simulink model "ModeStatAndRsp"  (R2018b)
settings: Solver=FixedStepDiscrete  StartTime=0.0  StopTime=10.0  FixedStep=0.01  RelTol=1e-3
undefined symbols (not defined in the file): c_RecvL, c_RecvLR, c_RecvR, IfVeSMSeStNumConfig, KeSMSbMdChime2Enable_Val, KeSMSbSRSPosNumConfig_Val, KeSMSuChmReqDurnTm_Val, KeSMSuChmReqIntlTm_Val, KeSMSuRspStatHldTm_Val, MdRspLocal1, MdTp1, ModeNum, PowerMode1, SrcReqTp1, srsconvert
libraries: RspLib x47, simulink x1
(part 7 of 8)

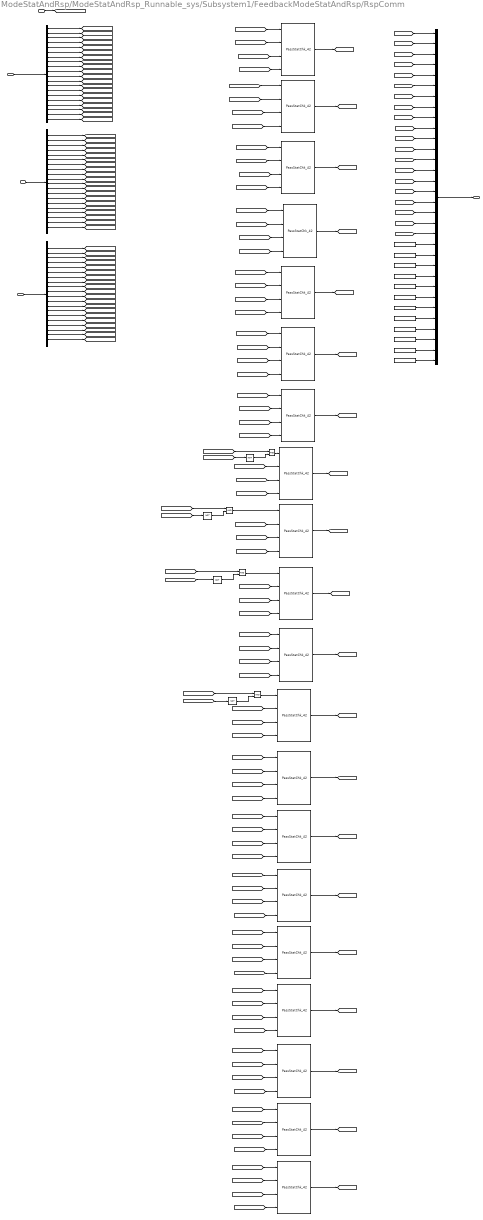
== system ModeStatAndRsp/ModeStatAndRsp_Runnable_sys/Subsystem1/FeedbackModeStatAndRsp/RspComm ==
  note: $0=No Status to Report; $1=Recall Successfully; $2=Recall UnSuccessfully_ Local Interrupt; $3=Recall UnSuccessfully_ Error; $4=Recall Ongoing; $5=Target Postion Already
  oModeStateBus : Inport
  oModeRsp : Inport  Port=2
  rspStateHldTm : Inport  Port=3
  IsArrivedAtTrgtPos : Inport  Port=4
  Bus Creator : BusCreator  Inputs=32
  Bus Selector : BusSelector  OutputSignals=Md1_En,Md2_En,Md3_En,Md4_En,Md5_En,Md6_En,Md7_En,Md8_En,Md9_En,Md10_En,Md11_En,Md12_En,Md13_En,Md14_En,Md15_En,Md16_En,Md17_En,Md18_En,Md19_En,Md20_En
  Bus Selector1 : BusSelector  OutputSignals=Md1TrgtPos,Md2TrgtPos,Md3TrgtPos,Md4TrgtPos,Md5TrgtPos,Md6TrgtPos,Md7TrgtPos,Md8TrgtPos,Md9TrgtPos,Md10TrgtPos,Md11TrgtPos,Md12TrgtPos,Md13TrgtPos,Md14TrgtPos,Md15TrgtPos,Md16TrgtPos,Md17TrgtPos,Md18TrgtPos,Md19TrgtPos,Md20TrgtPos
  Bus Selector2 : BusSelector  OutputSignals=Md1Rsp,Md2Rsp,Md3Rsp,Md4Rsp,Md5Rsp,Md6Rsp,Md7Rsp,Md8Rsp,Md9Rsp,Md10Rsp,Md11Rsp,Md12Rsp,Md13Rsp,Md14Rsp,Md15Rsp,Md16Rsp,Md17Rsp,Md18Rsp,Md19Rsp,Md20Rsp
  Constant{3..14} (12 alike) : Constant  Value=0  OutDataTypeStr=uint8
  Logical Operator{,1..2,6} (4 alike) : Logic  AllPortsSameDT=off  OutDataTypeStr=boolean
  Logical Operator{3..5,7} (4 alike) : Logic  Operator=NOT  AllPortsSameDT=off  OutDataTypeStr=boolean
  PassStatChk_Md{1..20} (20 alike) : RspLib/PassStatChk_42  SystemSampleTime=-1
  Rsp : Outport  VectorParamsAs1DForOutWhenUnconnected=on
  wires:
  rspStateHldTm/1 -> [rspStateHldTm]
  Bus Selector/11 -> [Md11_En]  "<Md11_En>"
  Bus Selector/12 -> [Md12_En]  "<Md12_En>"
  Bus Selector/13 -> [Md13_En]  "<Md13_En>"
  Bus Selector/6 -> [Md6_En]  "<Md6_En>"
  oModeRsp/1 -> Bus Selector2/1
  Bus Selector/14 -> [Md14_En]  "<Md14_En>"
  Bus Selector/3 -> [Md3_En]  "<Md3_En>"
  Bus Selector/10 -> [Md10_En]  "<Md10_En>"
  Bus Selector/8 -> [Md8_En]  "<Md8_En>"
  Bus Selector/1 -> [Md1_En]  "<Md1_En>"
  Bus Selector/15 -> [Md15_En]  "<Md15_En>"
  Bus Selector/7 -> [Md7_En]  "<Md7_En>"
  Bus Selector/2 -> [Md2_En]  "<Md2_En>"
  Bus Selector/4 -> [Md4_En]  "<Md4_En>"
  oModeStateBus/1 -> Bus Selector/1
  Bus Selector/9 -> [Md9_En]  "<Md9_En>"
  Bus Selector/5 -> [Md5_En]  "<Md5_En>"
  [rspStateHldTm] -> PassStatChk_Md1/2
  PassStatChk_Md1/1 -> [Md1RspOut]
  [rspStateHldTm] -> PassStatChk_Md4/2
  [rspStateHldTm] -> PassStatChk_Md3/2
  [rspStateHldTm] -> PassStatChk_Md8/2
  [rspStateHldTm] -> PassStatChk_Md9/2
  [Md1_En] -> PassStatChk_Md1/1
  [Md4_En] -> PassStatChk_Md4/1
  [Md3_En] -> PassStatChk_Md3/1
  [Md1Rsp] -> PassStatChk_Md1/3
  [Md4Rsp] -> PassStatChk_Md4/3
  [Md3Rsp] -> PassStatChk_Md3/3
  [Md8Rsp] -> PassStatChk_Md8/3
  [Md9Rsp] -> PassStatChk_Md9/3
  [Md2_En] -> PassStatChk_Md2/1
  [rspStateHldTm] -> PassStatChk_Md2/2
  [Md2Rsp] -> PassStatChk_Md2/3
  [Md5_En] -> PassStatChk_Md5/1
  [Md6_En] -> PassStatChk_Md6/1
  [Md7_En] -> PassStatChk_Md7/1
  [Md11_En] -> PassStatChk_Md11/1
  [Md13_En] -> PassStatChk_Md13/1
  [Md14_En] -> PassStatChk_Md14/1
  [Md15_En] -> PassStatChk_Md15/1
  [rspStateHldTm] -> PassStatChk_Md5/2
  [rspStateHldTm] -> PassStatChk_Md6/2
  [rspStateHldTm] -> PassStatChk_Md7/2
  [rspStateHldTm] -> PassStatChk_Md10/2
  [rspStateHldTm] -> PassStatChk_Md11/2
  [rspStateHldTm] -> PassStatChk_Md12/2
  [rspStateHldTm] -> PassStatChk_Md13/2
  [rspStateHldTm] -> PassStatChk_Md14/2
  [rspStateHldTm] -> PassStatChk_Md15/2
  [Md1RspOut] -> Bus Creator/1  "Md1RspOut"
  [Md12RspOut] -> Bus Creator/12  "Md12RspOut"
  [Md13RspOut] -> Bus Creator/13  "Md13RspOut"
  [Md14RspOut] -> Bus Creator/14  "Md14RspOut"
  [Md15RspOut] -> Bus Creator/15  "Md15RspOut"
  [Md8RspOut] -> Bus Creator/8  "Md8RspOut"
  [Md9RspOut] -> Bus Creator/9  "Md9RspOut"
  [Md10RspOut] -> Bus Creator/10  "Md10RspOut"
  [Md11RspOut] -> Bus Creator/11  "Md11RspOut"
  [Md7RspOut] -> Bus Creator/7  "Md7RspOut"
  [Md2RspOut] -> Bus Creator/2  "Md2RspOut"
  [Md3RspOut] -> Bus Creator/3  "Md3RspOut"
  [Md4RspOut] -> Bus Creator/4  "Md4RspOut"
  [Md5RspOut] -> Bus Creator/5  "Md5RspOut"
  [Md6RspOut] -> Bus Creator/6  "Md6RspOut"
  Bus Creator/1 -> Rsp/1
  Bus Selector2/1 -> [Md1Rsp]  "<Md1Rsp>"
  Bus Selector2/2 -> [Md2Rsp]  "<Md2Rsp>"
  Bus Selector2/3 -> [Md3Rsp]  "<Md3Rsp>"
  Bus Selector2/4 -> [Md4Rsp]  "<Md4Rsp>"
  Bus Selector2/5 -> [Md5Rsp]  "<Md5Rsp>"
  Bus Selector2/6 -> [Md6Rsp]  "<Md6Rsp>"
  Bus Selector2/7 -> [Md7Rsp]  "<Md7Rsp>"
  Bus Selector2/8 -> [Md8Rsp]  "<Md8Rsp>"
  Bus Selector2/9 -> [Md9Rsp]  "<Md9Rsp>"
  Bus Selector2/10 -> [Md10Rsp]  "<Md10Rsp>"
  Bus Selector2/11 -> [Md11Rsp]  "<Md11Rsp>"
  Bus Selector2/12 -> [Md12Rsp]  "<Md12Rsp>"
  Bus Selector2/13 -> [Md13Rsp]  "<Md13Rsp>"
  Bus Selector2/14 -> [Md14Rsp]  "<Md14Rsp>"
  Bus Selector2/15 -> [Md15Rsp]  "<Md15Rsp>"
  IsArrivedAtTrgtPos/1 -> Bus Selector1/1
  PassStatChk_Md2/1 -> [Md2RspOut]
  PassStatChk_Md3/1 -> [Md3RspOut]
  PassStatChk_Md4/1 -> [Md4RspOut]
  PassStatChk_Md5/1 -> [Md5RspOut]
  [Md5Rsp] -> PassStatChk_Md5/3
  [Md6Rsp] -> PassStatChk_Md6/3
  PassStatChk_Md6/1 -> [Md6RspOut]
  PassStatChk_Md7/1 -> [Md7RspOut]
  [Md7Rsp] -> PassStatChk_Md7/3
  [Md10Rsp] -> PassStatChk_Md10/3
  [Md11Rsp] -> PassStatChk_Md11/3
  PassStatChk_Md11/1 -> [Md11RspOut]
  [Md12Rsp] -> PassStatChk_Md12/3
  [Md13Rsp] -> PassStatChk_Md13/3
  PassStatChk_Md13/1 -> [Md13RspOut]
  [Md14Rsp] -> PassStatChk_Md14/3
  [Md15Rsp] -> PassStatChk_Md15/3
  PassStatChk_Md14/1 -> [Md14RspOut]
  PassStatChk_Md15/1 -> [Md15RspOut]
  Bus Selector1/1 -> [Md1TrgtPos]  "<Md1TrgtPos>"
  Bus Selector1/2 -> [Md2TrgtPos]  "<Md2TrgtPos>"
  Bus Selector1/3 -> [Md3TrgtPos]  "<Md3TrgtPos>"
  Bus Selector1/4 -> [Md4TrgtPos]  "<Md4TrgtPos>"
  Bus Selector1/5 -> [Md5TrgtPos]  "<Md5TrgtPos>"
  Bus Selector1/6 -> [Md6TrgtPos]  "<Md6TrgtPos>"
  Bus Selector1/7 -> [Md7TrgtPos]  "<Md7TrgtPos>"
  Bus Selector1/8 -> [Md8TrgtPos]  "<Md8TrgtPos>"
  Bus Selector1/9 -> [Md9TrgtPos]  "<Md9TrgtPos>"
  Bus Selector1/10 -> [Md10TrgtPos]  "<Md10TrgtPos>"
  Bus Selector1/11 -> [Md11TrgtPos]  "<Md11TrgtPos>"
  Bus Selector1/12 -> [Md12TrgtPos]  "<Md12TrgtPos>"
  Bus Selector1/13 -> [Md13TrgtPos]  "<Md13TrgtPos>"
  Bus Selector1/14 -> [Md14TrgtPos]  "<Md14TrgtPos>"
  Bus Selector1/15 -> [Md15TrgtPos]  "<Md15TrgtPos>"
  [Md1TrgtPos] -> PassStatChk_Md1/4
  [Md2TrgtPos] -> PassStatChk_Md2/4
  [Md3TrgtPos] -> PassStatChk_Md3/4
  [Md4TrgtPos] -> PassStatChk_Md4/4
  [Md6TrgtPos] -> PassStatChk_Md6/4
  [Md5TrgtPos] -> PassStatChk_Md5/4
  [Md7TrgtPos] -> PassStatChk_Md7/4
  [Md8TrgtPos] -> PassStatChk_Md8/4
  [Md9TrgtPos] -> PassStatChk_Md9/4
  [Md10TrgtPos] -> PassStatChk_Md10/4
  [Md11TrgtPos] -> PassStatChk_Md11/4
  [Md12TrgtPos] -> PassStatChk_Md12/4
  [Md13TrgtPos] -> PassStatChk_Md13/4
  [Md14TrgtPos] -> PassStatChk_Md14/4
  [Md15TrgtPos] -> PassStatChk_Md15/4
  PassStatChk_Md17/1 -> [Md17RspOut]
  PassStatChk_Md16/1 -> [Md16RspOut]
  [Md16Rsp] -> PassStatChk_Md16/3
  [rspStateHldTm] -> PassStatChk_Md16/2
  [Md16_En] -> PassStatChk_Md16/1
  [Md16TrgtPos] -> PassStatChk_Md16/4
  [Md17_En] -> PassStatChk_Md17/1
  [rspStateHldTm] -> PassStatChk_Md17/2
  [Md17Rsp] -> PassStatChk_Md17/3
  [Md17TrgtPos] -> PassStatChk_Md17/4
  Bus Selector2/16 -> [Md16Rsp]  "<Md16Rsp>"
  Bus Selector2/17 -> [Md17Rsp]  "<Md17Rsp>"
  Bus Selector1/17 -> [Md17TrgtPos]  "<Md17TrgtPos>"
  Bus Selector1/16 -> [Md16TrgtPos]  "<Md16TrgtPos>"
  Bus Selector/16 -> [Md16_En]  "<Md16_En>"
  Bus Selector/17 -> [Md17_En]  "<Md17_En>"
  [Md16RspOut] -> Bus Creator/16  "Md16RspOut"
  [Md17RspOut] -> Bus Creator/17  "Md17RspOut"
  [Md18RspOut] -> Bus Creator/18  "Md18RspOut"
  [Md19RspOut] -> Bus Creator/19  "Md19RspOut"
  [Md20RspOut] -> Bus Creator/20  "Md20RspOut"
  Constant3/1 -> Bus Creator/21  "Md21RspOut"
  Constant4/1 -> Bus Creator/22  "Md22RspOut"
  Constant5/1 -> Bus Creator/23  "Md23RspOut"
  Constant6/1 -> Bus Creator/24  "Md24RspOut"
  Constant7/1 -> Bus Creator/25  "Md25RspOut"
  Constant8/1 -> Bus Creator/26  "Md26RspOut"
  Constant9/1 -> Bus Creator/27  "Md27RspOut"
  Constant10/1 -> Bus Creator/28  "Md28RspOut"
  Constant11/1 -> Bus Creator/29  "Md29RspOut"
  Constant14/1 -> Bus Creator/30  "Md30RspOut"
  Constant12/1 -> Bus Creator/31  "Md31RspOut"
  Constant13/1 -> Bus Creator/32  "Md32RspOut"
  [Md3_En] -> Logical Operator5/1
  PassStatChk_Md8/1 -> [Md8RspOut]
  PassStatChk_Md9/1 -> [Md9RspOut]
  PassStatChk_Md12/1 -> [Md12RspOut]
  Logical Operator/1 -> PassStatChk_Md8/1
  Logical Operator5/1 -> Logical Operator/2
  [Md8_En] -> Logical Operator/1
  Logical Operator3/1 -> Logical Operator2/2
  [Md3_En] -> Logical Operator3/1
  [Md9_En] -> Logical Operator2/1
  Logical Operator2/1 -> PassStatChk_Md9/1
  [Md10_En] -> Logical Operator6/1
  [Md2_En] -> Logical Operator7/1
  Logical Operator7/1 -> Logical Operator6/2
  Logical Operator6/1 -> PassStatChk_Md10/1
  PassStatChk_Md10/1 -> [Md10RspOut]
  Logical Operator4/1 -> Logical Operator1/2
  [Md2_En] -> Logical Operator4/1
  Logical Operator1/1 -> PassStatChk_Md12/1
  [Md12_En] -> Logical Operator1/1
  [Md18TrgtPos] -> PassStatChk_Md18/4
  [Md18Rsp] -> PassStatChk_Md18/3
  [rspStateHldTm] -> PassStatChk_Md18/2
  [Md18_En] -> PassStatChk_Md18/1
  PassStatChk_Md18/1 -> [Md18RspOut]
  PassStatChk_Md19/1 -> [Md19RspOut]
  [Md19_En] -> PassStatChk_Md19/1
  [rspStateHldTm] -> PassStatChk_Md19/2
  [Md19Rsp] -> PassStatChk_Md19/3
  [Md19TrgtPos] -> PassStatChk_Md19/4
  [Md20TrgtPos] -> PassStatChk_Md20/4
  [Md20Rsp] -> PassStatChk_Md20/3
  [rspStateHldTm] -> PassStatChk_Md20/2
  [Md20_En] -> PassStatChk_Md20/1
  PassStatChk_Md20/1 -> [Md20RspOut]
  Bus Selector/18 -> [Md18_En]  "<Md18_En>"
  Bus Selector/19 -> [Md19_En]  "<Md19_En>"
  Bus Selector/20 -> [Md20_En]  "<Md20_En>"
  Bus Selector2/18 -> [Md18Rsp]  "<Md18Rsp>"
  Bus Selector2/19 -> [Md19Rsp]  "<Md19Rsp>"
  Bus Selector2/20 -> [Md20Rsp]  "<Md20Rsp>"
  Bus Selector1/18 -> [Md18TrgtPos]  "<Md18TrgtPos>"
  Bus Selector1/19 -> [Md19TrgtPos]  "<Md19TrgtPos>"
  Bus Selector1/20 -> [Md20TrgtPos]  "<Md20TrgtPos>"

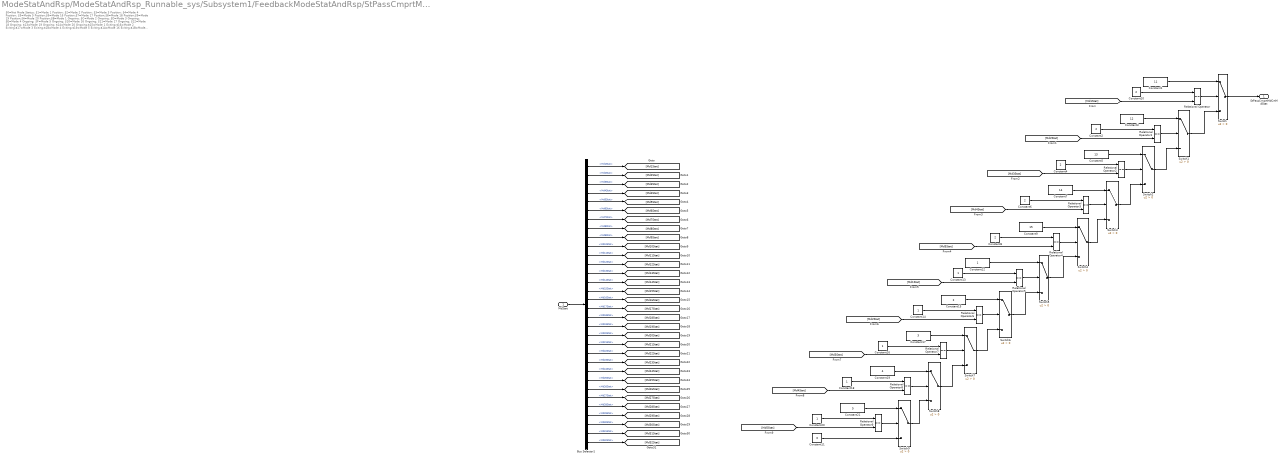
== system ModeStatAndRsp/ModeStatAndRsp_Runnable_sys/Subsystem1/FeedbackModeStatAndRsp/StPassCmprtMdCrtMdStat_3A6 ==
  note: $0=Not Mode Status; $1=Mode 1 Position; $2=Mode 2 Position; $3=Mode 3 Position; $4=Mode 4 Position; $5=Mode 5 Position;$6=Mode 16 Position;$7=Mode 17 Position;$8=Mode 18 Position;$9=Mode 19 Position;$A=Mode 20 Position;$B=Mode 1 Ongoing; $C=Mode 2 Ongoing; $D=Mode 3 Ongoing; $E=Mode 4 Ongoing; $F=Mode 5 Ongoing; $10=Mode 16 Ongoing; $11=Mode 17 Ongoing; $12=Mode 18 Ongoing; $13=Mode 19 Ongoing; $14=Mode 20 Ongoing;$15=Mode 1 Exiting;$16=Mode 2 Exiting;$17=Mode 3 Exiting;$18=Mode 4 Exiting;$19=Mode 5 Exiting;$1A=Mode 16 Exiting;$1B=Mode 17 Exiting;$1C=Mode 18 Exiting;$1D=Mode 19 Exiting;$1E=Mode 20 Exiting;
  MdStat : Inport
  Bus Selector1 : BusSelector  OutputSignals=Md1Stat,Md2Stat,Md3Stat,Md4Stat,Md5Stat,Md6Stat,Md7Stat,Md8Stat,Md9Stat,Md10Stat,Md11Stat,Md12Stat,Md13Stat,Md14Stat,Md15Stat,Md16Stat,Md17Stat,Md18Stat,Md19Stat,Md20Stat,Md21Stat,Md22Stat,Md23Stat,Md24Stat,Md25Stat,Md26Stat,Md27Stat,Md28Stat,Md29Stat,Md30Stat,Md31Stat,Md32Stat
  Constant1 : Constant  Value=11  OutDataTypeStr=uint8
  Constant{2,4,6,8,10,15} (6 alike) : Constant  Value=2  OutDataTypeStr=uint8
  Constant11 : Constant  Value=0  OutDataTypeStr=uint8
  Constant{12..14,16,18,20} (6 alike) : Constant  OutDataTypeStr=uint8
  Constant17 : Constant  Value=3  OutDataTypeStr=uint8
  Constant19 : Constant  Value=4  OutDataTypeStr=uint8
  Constant21 : Constant  Value=5  OutDataTypeStr=uint8
  Constant3 : Constant  Value=12  OutDataTypeStr=uint8
  Constant5 : Constant  Value=13  OutDataTypeStr=uint8
  Constant7 : Constant  Value=14  OutDataTypeStr=uint8
  Constant9 : Constant  Value=15  OutDataTypeStr=uint8
  Relational Operator{,1..9} (10 alike) : RelationalOperator  Operator===  OutDataTypeStr=boolean  RndMeth=Simplest
  Switch{,1..9} (10 alike) : Switch  Criteria=u2 > Threshold
  StPassCmprtMdCrtMdStat : Outport
  wires:
  Switch/1 -> StPassCmprtMdCrtMdStat/1
  MdStat/1 -> Bus Selector1/1
  Bus Selector1/30 -> [Md30Stat]  "<Md30Stat>"
  Bus Selector1/29 -> [Md29Stat]  "<Md29Stat>"
  Bus Selector1/27 -> [Md27Stat]  "<Md27Stat>"
  Bus Selector1/24 -> [Md24Stat]  "<Md24Stat>"
  Bus Selector1/22 -> [Md22Stat]  "<Md22Stat>"
  Bus Selector1/26 -> [Md26Stat]  "<Md26Stat>"
  Bus Selector1/25 -> [Md25Stat]  "<Md25Stat>"
  Bus Selector1/32 -> [Md32Stat]  "<Md32Stat>"
  Bus Selector1/23 -> [Md23Stat]  "<Md23Stat>"
  Bus Selector1/20 -> [Md20Stat]  "<Md20Stat>"
  Bus Selector1/31 -> [Md31Stat]  "<Md31Stat>"
  Bus Selector1/19 -> [Md19Stat]  "<Md19Stat>"
  Bus Selector1/18 -> [Md18Stat]  "<Md18Stat>"
  Bus Selector1/21 -> [Md21Stat]  "<Md21Stat>"
  Bus Selector1/28 -> [Md28Stat]  "<Md28Stat>"
  Bus Selector1/14 -> [Md14Stat]  "<Md14Stat>"
  Bus Selector1/17 -> [Md17Stat]  "<Md17Stat>"
  Bus Selector1/15 -> [Md15Stat]  "<Md15Stat>"
  Bus Selector1/12 -> [Md12Stat]  "<Md12Stat>"
  Bus Selector1/9 -> [Md9Stat]  "<Md9Stat>"
  Bus Selector1/10 -> [Md10Stat]  "<Md10Stat>"
  Bus Selector1/6 -> [Md6Stat]  "<Md6Stat>"
  Bus Selector1/5 -> [Md5Stat]  "<Md5Stat>"
  Bus Selector1/11 -> [Md11Stat]  "<Md11Stat>"
  Bus Selector1/13 -> [Md13Stat]  "<Md13Stat>"
  Bus Selector1/4 -> [Md4Stat]  "<Md4Stat>"
  Bus Selector1/8 -> [Md8Stat]  "<Md8Stat>"
  Bus Selector1/2 -> [Md2Stat]  "<Md2Stat>"
  Bus Selector1/1 -> [Md1Stat]  "<Md1Stat>"
  Bus Selector1/3 -> [Md3Stat]  "<Md3Stat>"
  Bus Selector1/7 -> [Md7Stat]  "<Md7Stat>"
  Bus Selector1/16 -> [Md16Stat]  "<Md16Stat>"
  [Md1Stat] -> Relational Operator/2
  Constant10/1 -> Relational Operator/1
  Relational Operator/1 -> Switch/2
  Constant1/1 -> Switch/1
  Switch1/1 -> Switch/3
  Relational Operator1/1 -> Switch1/2
  Constant2/1 -> Relational Operator1/1
  [Md2Stat] -> Relational Operator1/2
  Constant3/1 -> Switch1/1
  Constant5/1 -> Switch2/1
  [Md3Stat] -> Relational Operator2/2
  Constant4/1 -> Relational Operator2/1
  Relational Operator2/1 -> Switch2/2
  Switch2/1 -> Switch1/3
  Switch3/1 -> Switch2/3
  Relational Operator3/1 -> Switch3/2
  Constant6/1 -> Relational Operator3/1
  [Md4Stat] -> Relational Operator3/2
  Constant7/1 -> Switch3/1
  Constant9/1 -> Switch4/1
  [Md5Stat] -> Relational Operator4/2
  Constant8/1 -> Relational Operator4/1
  Relational Operator4/1 -> Switch4/2
  Switch4/1 -> Switch3/3
  Switch9/1 -> Switch8/3
  Relational Operator9/1 -> Switch9/2
  Constant20/1 -> Relational Operator9/1
  [Md5Stat] -> Relational Operator9/2
  Constant21/1 -> Switch9/1
  Constant19/1 -> Switch8/1
  [Md4Stat] -> Relational Operator8/2
  Constant18/1 -> Relational Operator8/1
  Relational Operator8/1 -> Switch8/2
  Switch8/1 -> Switch7/3
  Switch7/1 -> Switch6/3
  Relational Operator7/1 -> Switch7/2
  Constant16/1 -> Relational Operator7/1
  [Md3Stat] -> Relational Operator7/2
  Constant17/1 -> Switch7/1
  Constant15/1 -> Switch6/1
  [Md2Stat] -> Relational Operator6/2
  Constant14/1 -> Relational Operator6/1
  Relational Operator6/1 -> Switch6/2
  Switch6/1 -> Switch5/3
  Constant12/1 -> Switch5/1
  Relational Operator5/1 -> Switch5/2
  Constant13/1 -> Relational Operator5/1
  [Md1Stat] -> Relational Operator5/2
  Switch5/1 -> Switch4/3
  Constant11/1 -> Switch9/3

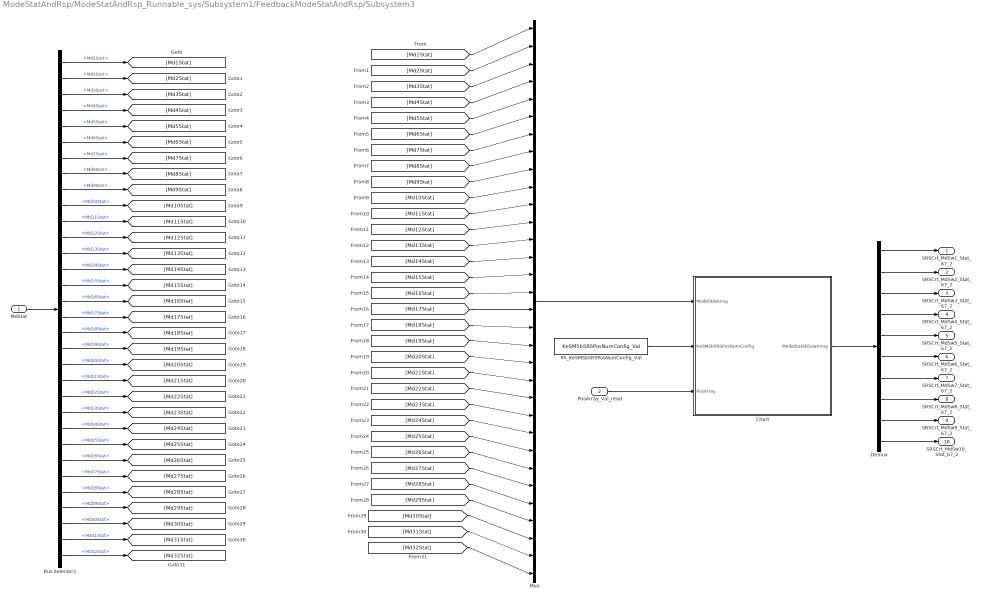
== system ModeStatAndRsp/ModeStatAndRsp_Runnable_sys/Subsystem1/FeedbackModeStatAndRsp/Subsystem3 ==
  MdStat : Inport
  PosArray_Val_read : Inport  Port=2
  Bus Selector1 : BusSelector  OutputSignals=Md1Stat,Md2Stat,Md3Stat,Md4Stat,Md5Stat,Md6Stat,Md7Stat,Md8Stat,Md9Stat,Md10Stat,Md11Stat,Md12Stat,Md13Stat,Md14Stat,Md15Stat,Md16Stat,Md17Stat,Md18Stat,Md19Stat,Md20Stat,Md21Stat,Md22Stat,Md23Stat,Md24Stat,Md25Stat,Md26Stat,Md27Stat,Md28Stat,Md29Stat,Md30Stat,Md31Stat,Md32Stat
  Chart : Stateflow chart  TreatAsAtomicUnit=on
  Demux : Demux  Outputs=10
  Mux : Mux  Inputs=32
  PA_KeSMSbSRSPosNumConfig_Val : Constant  Value=KeSMSbSRSPosNumConfig_Val
  SRSCrt_MdSw1_Stat_67_2 : Outport
  SRSCrt_MdSw2_Stat_67_2 : Outport  Port=2
  SRSCrt_MdSw3_Stat_67_2 : Outport  Port=3
  SRSCrt_MdSw4_Stat_67_2 : Outport  Port=4
  SRSCrt_MdSw5_Stat_67_2 : Outport  Port=5
  SRSCrt_MdSw6_Stat_67_2 : Outport  Port=6
  SRSCrt_MdSw7_Stat_67_2 : Outport  Port=7
  SRSCrt_MdSw8_Stat_67_2 : Outport  Port=8
  SRSCrt_MdSw9_Stat_67_2 : Outport  Port=9
  SRSCrt_MdSw10_Stat_67_2 : Outport  Port=10
  wires:
  Demux/5 -> SRSCrt_MdSw5_Stat_67_2/1
  Demux/6 -> SRSCrt_MdSw6_Stat_67_2/1
  Demux/7 -> SRSCrt_MdSw7_Stat_67_2/1
  Demux/8 -> SRSCrt_MdSw8_Stat_67_2/1
  Demux/9 -> SRSCrt_MdSw9_Stat_67_2/1
  Demux/10 -> SRSCrt_MdSw10_Stat_67_2/1
  Bus Selector1/10 -> [Md10Stat]  "<Md10Stat>"
  Bus Selector1/1 -> [Md1Stat]  "<Md1Stat>"
  Bus Selector1/9 -> [Md9Stat]  "<Md9Stat>"
  Bus Selector1/5 -> [Md5Stat]  "<Md5Stat>"
  Bus Selector1/14 -> [Md14Stat]  "<Md14Stat>"
  Bus Selector1/15 -> [Md15Stat]  "<Md15Stat>"
  Bus Selector1/4 -> [Md4Stat]  "<Md4Stat>"
  Bus Selector1/30 -> [Md30Stat]  "<Md30Stat>"
  Bus Selector1/11 -> [Md11Stat]  "<Md11Stat>"
  Bus Selector1/29 -> [Md29Stat]  "<Md29Stat>"
  Bus Selector1/12 -> [Md12Stat]  "<Md12Stat>"
  Bus Selector1/2 -> [Md2Stat]  "<Md2Stat>"
  Bus Selector1/25 -> [Md25Stat]  "<Md25Stat>"
  Bus Selector1/6 -> [Md6Stat]  "<Md6Stat>"
  Bus Selector1/8 -> [Md8Stat]  "<Md8Stat>"
  Bus Selector1/3 -> [Md3Stat]  "<Md3Stat>"
  MdStat/1 -> Bus Selector1/1
  Bus Selector1/7 -> [Md7Stat]  "<Md7Stat>"
  Bus Selector1/27 -> [Md27Stat]  "<Md27Stat>"
  Bus Selector1/22 -> [Md22Stat]  "<Md22Stat>"
  Bus Selector1/21 -> [Md21Stat]  "<Md21Stat>"
  Bus Selector1/20 -> [Md20Stat]  "<Md20Stat>"
  Bus Selector1/13 -> [Md13Stat]  "<Md13Stat>"
  Bus Selector1/17 -> [Md17Stat]  "<Md17Stat>"
  Bus Selector1/18 -> [Md18Stat]  "<Md18Stat>"
  Bus Selector1/24 -> [Md24Stat]  "<Md24Stat>"
  Bus Selector1/19 -> [Md19Stat]  "<Md19Stat>"
  Bus Selector1/26 -> [Md26Stat]  "<Md26Stat>"
  Bus Selector1/31 -> [Md31Stat]  "<Md31Stat>"
  Bus Selector1/16 -> [Md16Stat]  "<Md16Stat>"
  Bus Selector1/23 -> [Md23Stat]  "<Md23Stat>"
  Bus Selector1/28 -> [Md28Stat]  "<Md28Stat>"
  Bus Selector1/32 -> [Md32Stat]  "<Md32Stat>"
  Demux/1 -> SRSCrt_MdSw1_Stat_67_2/1
  Demux/2 -> SRSCrt_MdSw2_Stat_67_2/1
  Demux/3 -> SRSCrt_MdSw3_Stat_67_2/1
  Demux/4 -> SRSCrt_MdSw4_Stat_67_2/1
  [Md1Stat] -> Mux/1
  [Md2Stat] -> Mux/2
  [Md26Stat] -> Mux/26
  [Md27Stat] -> Mux/27
  [Md28Stat] -> Mux/28
  [Md23Stat] -> Mux/23
  [Md24Stat] -> Mux/24
  [Md25Stat] -> Mux/25
  [Md29Stat] -> Mux/29
  [Md30Stat] -> Mux/30
  [Md5Stat] -> Mux/5
  [Md6Stat] -> Mux/6
  [Md13Stat] -> Mux/13
  [Md14Stat] -> Mux/14
  [Md20Stat] -> Mux/20
  [Md21Stat] -> Mux/21
  [Md22Stat] -> Mux/22
  [Md7Stat] -> Mux/7
  [Md10Stat] -> Mux/10
  [Md11Stat] -> Mux/11
  [Md12Stat] -> Mux/12
  [Md15Stat] -> Mux/15
  [Md16Stat] -> Mux/16
  [Md17Stat] -> Mux/17
  [Md19Stat] -> Mux/19
  [Md31Stat] -> Mux/31
  [Md32Stat] -> Mux/32
  [Md8Stat] -> Mux/8
  [Md9Stat] -> Mux/9
  [Md18Stat] -> Mux/18
  Mux/1 -> Chart/1(ModeStatArray)
  PA_KeSMSbSRSPosNumConfig_Val/1 -> Chart/2(KeSMSbSRSPosNumConfig)
  Chart/1(ModeStatSRSswArray) -> Demux/1
  PosArray_Val_read/1 -> Chart/3(PosArray)
  [Md4Stat] -> Mux/4
  [Md3Stat] -> Mux/3

== system ModeStatAndRsp/ModeStatAndRsp_Runnable_sys/Subsystem1/Subsystem/HasChangeToTrue ==
  In1 : Inport
  AND : Logic  AllPortsSameDT=off  OutDataTypeStr=boolean
  Constant : Constant  OutDataTypeStr=boolean
  Relational Operator : RelationalOperator  Operator=~=  OutDataTypeStr=boolean  RndMeth=Simplest
  Relational Operator1 : RelationalOperator  Operator===  OutDataTypeStr=boolean  RndMeth=Simplest
  Unit Delay : UnitDelay  SampleTime=-1
  Out1 : Outport
  wires:
  In1/1 -> Relational Operator1/2, Relational Operator/1, Unit Delay/1
  Unit Delay/1 -> Relational Operator/2
  Relational Operator/1 -> AND/2
  Constant/1 -> Relational Operator1/1
  Relational Operator1/1 -> AND/1
  AND/1 -> Out1/1

== system ModeStatAndRsp/ModeStatAndRsp_Runnable_sys/Subsystem1/Subsystem/HasChangeToTrue1 ==
  In1 : Inport
  AND : Logic  AllPortsSameDT=off  OutDataTypeStr=boolean
  Constant : Constant  OutDataTypeStr=boolean
  Relational Operator : RelationalOperator  Operator=~=  OutDataTypeStr=boolean  RndMeth=Simplest
  Relational Operator1 : RelationalOperator  Operator===  OutDataTypeStr=boolean  RndMeth=Simplest
  Unit Delay : UnitDelay  SampleTime=-1
  Out1 : Outport
  wires:
  AND/1 -> Out1/1
  Relational Operator1/1 -> AND/1
  Constant/1 -> Relational Operator1/1
  Relational Operator/1 -> AND/2
  Unit Delay/1 -> Relational Operator/2
  In1/1 -> Unit Delay/1, Relational Operator/1, Relational Operator1/2

== system ModeStatAndRsp/ModeStatAndRsp_Runnable_sys/Subsystem1/Subsystem/HasChangeToTrue10 ==
  In1 : Inport
  AND : Logic  AllPortsSameDT=off  OutDataTypeStr=boolean
  Constant : Constant  OutDataTypeStr=boolean
  Relational Operator : RelationalOperator  Operator=~=  OutDataTypeStr=boolean  RndMeth=Simplest
  Relational Operator1 : RelationalOperator  Operator===  OutDataTypeStr=boolean  RndMeth=Simplest
  Unit Delay : UnitDelay  SampleTime=-1
  Out1 : Outport
  wires:
  AND/1 -> Out1/1
  Relational Operator1/1 -> AND/1
  Constant/1 -> Relational Operator1/1
  Relational Operator/1 -> AND/2
  Unit Delay/1 -> Relational Operator/2
  In1/1 -> Unit Delay/1, Relational Operator/1, Relational Operator1/2

== system ModeStatAndRsp/ModeStatAndRsp_Runnable_sys/Subsystem1/Subsystem/HasChangeToTrue11 ==
  In1 : Inport
  AND : Logic  AllPortsSameDT=off  OutDataTypeStr=boolean
  Constant : Constant  OutDataTypeStr=boolean
  Relational Operator : RelationalOperator  Operator=~=  OutDataTypeStr=boolean  RndMeth=Simplest
  Relational Operator1 : RelationalOperator  Operator===  OutDataTypeStr=boolean  RndMeth=Simplest
  Unit Delay : UnitDelay  SampleTime=-1
  Out1 : Outport
  wires:
  AND/1 -> Out1/1
  Relational Operator1/1 -> AND/1
  Constant/1 -> Relational Operator1/1
  Relational Operator/1 -> AND/2
  Unit Delay/1 -> Relational Operator/2
  In1/1 -> Unit Delay/1, Relational Operator/1, Relational Operator1/2

== system ModeStatAndRsp/ModeStatAndRsp_Runnable_sys/Subsystem1/Subsystem/HasChangeToTrue12 ==
  In1 : Inport
  AND : Logic  AllPortsSameDT=off  OutDataTypeStr=boolean
  Constant : Constant  OutDataTypeStr=boolean
  Relational Operator : RelationalOperator  Operator=~=  OutDataTypeStr=boolean  RndMeth=Simplest
  Relational Operator1 : RelationalOperator  Operator===  OutDataTypeStr=boolean  RndMeth=Simplest
  Unit Delay : UnitDelay  SampleTime=-1
  Out1 : Outport
  wires:
  AND/1 -> Out1/1
  Relational Operator1/1 -> AND/1
  Constant/1 -> Relational Operator1/1
  Relational Operator/1 -> AND/2
  Unit Delay/1 -> Relational Operator/2
  In1/1 -> Unit Delay/1, Relational Operator/1, Relational Operator1/2

== system ModeStatAndRsp/ModeStatAndRsp_Runnable_sys/Subsystem1/Subsystem/HasChangeToTrue13 ==
  In1 : Inport
  AND : Logic  AllPortsSameDT=off  OutDataTypeStr=boolean
  Constant : Constant  OutDataTypeStr=boolean
  Relational Operator : RelationalOperator  Operator=~=  OutDataTypeStr=boolean  RndMeth=Simplest
  Relational Operator1 : RelationalOperator  Operator===  OutDataTypeStr=boolean  RndMeth=Simplest
  Unit Delay : UnitDelay  SampleTime=-1
  Out1 : Outport
  wires:
  AND/1 -> Out1/1
  Relational Operator1/1 -> AND/1
  Constant/1 -> Relational Operator1/1
  Relational Operator/1 -> AND/2
  Unit Delay/1 -> Relational Operator/2
  In1/1 -> Unit Delay/1, Relational Operator/1, Relational Operator1/2

== system ModeStatAndRsp/ModeStatAndRsp_Runnable_sys/Subsystem1/Subsystem/HasChangeToTrue14 ==
  In1 : Inport
  AND : Logic  AllPortsSameDT=off  OutDataTypeStr=boolean
  Constant : Constant  OutDataTypeStr=boolean
  Relational Operator : RelationalOperator  Operator=~=  OutDataTypeStr=boolean  RndMeth=Simplest
  Relational Operator1 : RelationalOperator  Operator===  OutDataTypeStr=boolean  RndMeth=Simplest
  Unit Delay : UnitDelay  SampleTime=-1
  Out1 : Outport
  wires:
  AND/1 -> Out1/1
  Relational Operator1/1 -> AND/1
  Constant/1 -> Relational Operator1/1
  Relational Operator/1 -> AND/2
  Unit Delay/1 -> Relational Operator/2
  In1/1 -> Unit Delay/1, Relational Operator/1, Relational Operator1/2

== system ModeStatAndRsp/ModeStatAndRsp_Runnable_sys/Subsystem1/Subsystem/HasChangeToTrue15 ==
  In1 : Inport
  AND : Logic  AllPortsSameDT=off  OutDataTypeStr=boolean
  Constant : Constant  OutDataTypeStr=boolean
  Relational Operator : RelationalOperator  Operator=~=  OutDataTypeStr=boolean  RndMeth=Simplest
  Relational Operator1 : RelationalOperator  Operator===  OutDataTypeStr=boolean  RndMeth=Simplest
  Unit Delay : UnitDelay  SampleTime=-1
  Out1 : Outport
  wires:
  In1/1 -> Relational Operator1/2, Relational Operator/1, Unit Delay/1
  Unit Delay/1 -> Relational Operator/2
  Relational Operator/1 -> AND/2
  Constant/1 -> Relational Operator1/1
  Relational Operator1/1 -> AND/1
  AND/1 -> Out1/1

== system ModeStatAndRsp/ModeStatAndRsp_Runnable_sys/Subsystem1/Subsystem/HasChangeToTrue16 ==
  In1 : Inport
  AND : Logic  AllPortsSameDT=off  OutDataTypeStr=boolean
  Constant : Constant  OutDataTypeStr=boolean
  Relational Operator : RelationalOperator  Operator=~=  OutDataTypeStr=boolean  RndMeth=Simplest
  Relational Operator1 : RelationalOperator  Operator===  OutDataTypeStr=boolean  RndMeth=Simplest
  Unit Delay : UnitDelay  SampleTime=-1
  Out1 : Outport
  wires:
  AND/1 -> Out1/1
  Relational Operator1/1 -> AND/1
  Constant/1 -> Relational Operator1/1
  Relational Operator/1 -> AND/2
  Unit Delay/1 -> Relational Operator/2
  In1/1 -> Unit Delay/1, Relational Operator/1, Relational Operator1/2

== system ModeStatAndRsp/ModeStatAndRsp_Runnable_sys/Subsystem1/Subsystem/HasChangeToTrue17 ==
  In1 : Inport
  AND : Logic  AllPortsSameDT=off  OutDataTypeStr=boolean
  Constant : Constant  OutDataTypeStr=boolean
  Relational Operator : RelationalOperator  Operator=~=  OutDataTypeStr=boolean  RndMeth=Simplest
  Relational Operator1 : RelationalOperator  Operator===  OutDataTypeStr=boolean  RndMeth=Simplest
  Unit Delay : UnitDelay  SampleTime=-1
  Out1 : Outport
  wires:
  In1/1 -> Relational Operator1/2, Relational Operator/1, Unit Delay/1
  Unit Delay/1 -> Relational Operator/2
  Relational Operator/1 -> AND/2
  Constant/1 -> Relational Operator1/1
  Relational Operator1/1 -> AND/1
  AND/1 -> Out1/1

== system ModeStatAndRsp/ModeStatAndRsp_Runnable_sys/Subsystem1/Subsystem/HasChangeToTrue18 ==
  In1 : Inport
  AND : Logic  AllPortsSameDT=off  OutDataTypeStr=boolean
  Constant : Constant  OutDataTypeStr=boolean
  Relational Operator : RelationalOperator  Operator=~=  OutDataTypeStr=boolean  RndMeth=Simplest
  Relational Operator1 : RelationalOperator  Operator===  OutDataTypeStr=boolean  RndMeth=Simplest
  Unit Delay : UnitDelay  SampleTime=-1
  Out1 : Outport
  wires:
  AND/1 -> Out1/1
  Relational Operator1/1 -> AND/1
  Constant/1 -> Relational Operator1/1
  Relational Operator/1 -> AND/2
  Unit Delay/1 -> Relational Operator/2
  In1/1 -> Unit Delay/1, Relational Operator/1, Relational Operator1/2

== system ModeStatAndRsp/ModeStatAndRsp_Runnable_sys/Subsystem1/Subsystem/HasChangeToTrue19 ==
  In1 : Inport
  AND : Logic  AllPortsSameDT=off  OutDataTypeStr=boolean
  Constant : Constant  OutDataTypeStr=boolean
  Relational Operator : RelationalOperator  Operator=~=  OutDataTypeStr=boolean  RndMeth=Simplest
  Relational Operator1 : RelationalOperator  Operator===  OutDataTypeStr=boolean  RndMeth=Simplest
  Unit Delay : UnitDelay  SampleTime=-1
  Out1 : Outport
  wires:
  In1/1 -> Relational Operator1/2, Relational Operator/1, Unit Delay/1
  Unit Delay/1 -> Relational Operator/2
  Relational Operator/1 -> AND/2
  Constant/1 -> Relational Operator1/1
  Relational Operator1/1 -> AND/1
  AND/1 -> Out1/1

== system ModeStatAndRsp/ModeStatAndRsp_Runnable_sys/Subsystem1/Subsystem/HasChangeToTrue2 ==
  In1 : Inport
  AND : Logic  AllPortsSameDT=off  OutDataTypeStr=boolean
  Constant : Constant  OutDataTypeStr=boolean
  Relational Operator : RelationalOperator  Operator=~=  OutDataTypeStr=boolean  RndMeth=Simplest
  Relational Operator1 : RelationalOperator  Operator===  OutDataTypeStr=boolean  RndMeth=Simplest
  Unit Delay : UnitDelay  SampleTime=-1
  Out1 : Outport
  wires:
  In1/1 -> Relational Operator1/2, Relational Operator/1, Unit Delay/1
  Unit Delay/1 -> Relational Operator/2
  Relational Operator/1 -> AND/2
  Constant/1 -> Relational Operator1/1
  Relational Operator1/1 -> AND/1
  AND/1 -> Out1/1

== system ModeStatAndRsp/ModeStatAndRsp_Runnable_sys/Subsystem1/Subsystem/HasChangeToTrue3 ==
  In1 : Inport
  AND : Logic  AllPortsSameDT=off  OutDataTypeStr=boolean
  Constant : Constant  OutDataTypeStr=boolean
  Relational Operator : RelationalOperator  Operator=~=  OutDataTypeStr=boolean  RndMeth=Simplest
  Relational Operator1 : RelationalOperator  Operator===  OutDataTypeStr=boolean  RndMeth=Simplest
  Unit Delay : UnitDelay  SampleTime=-1
  Out1 : Outport
  wires:
  AND/1 -> Out1/1
  Relational Operator1/1 -> AND/1
  Constant/1 -> Relational Operator1/1
  Relational Operator/1 -> AND/2
  Unit Delay/1 -> Relational Operator/2
  In1/1 -> Unit Delay/1, Relational Operator/1, Relational Operator1/2

== system ModeStatAndRsp/ModeStatAndRsp_Runnable_sys/Subsystem1/Subsystem/HasChangeToTrue4 ==
  In1 : Inport
  AND : Logic  AllPortsSameDT=off  OutDataTypeStr=boolean
  Constant : Constant  OutDataTypeStr=boolean
  Relational Operator : RelationalOperator  Operator=~=  OutDataTypeStr=boolean  RndMeth=Simplest
  Relational Operator1 : RelationalOperator  Operator===  OutDataTypeStr=boolean  RndMeth=Simplest
  Unit Delay : UnitDelay  SampleTime=-1
  Out1 : Outport
  wires:
  In1/1 -> Relational Operator1/2, Relational Operator/1, Unit Delay/1
  Unit Delay/1 -> Relational Operator/2
  Relational Operator/1 -> AND/2
  Constant/1 -> Relational Operator1/1
  Relational Operator1/1 -> AND/1
  AND/1 -> Out1/1

== system ModeStatAndRsp/ModeStatAndRsp_Runnable_sys/Subsystem1/Subsystem/HasChangeToTrue5 ==
  In1 : Inport
  AND : Logic  AllPortsSameDT=off  OutDataTypeStr=boolean
  Constant : Constant  OutDataTypeStr=boolean
  Relational Operator : RelationalOperator  Operator=~=  OutDataTypeStr=boolean  RndMeth=Simplest
  Relational Operator1 : RelationalOperator  Operator===  OutDataTypeStr=boolean  RndMeth=Simplest
  Unit Delay : UnitDelay  SampleTime=-1
  Out1 : Outport
  wires:
  AND/1 -> Out1/1
  Relational Operator1/1 -> AND/1
  Constant/1 -> Relational Operator1/1
  Relational Operator/1 -> AND/2
  Unit Delay/1 -> Relational Operator/2
  In1/1 -> Unit Delay/1, Relational Operator/1, Relational Operator1/2

== system ModeStatAndRsp/ModeStatAndRsp_Runnable_sys/Subsystem1/Subsystem/HasChangeToTrue6 ==
  In1 : Inport
  AND : Logic  AllPortsSameDT=off  OutDataTypeStr=boolean
  Constant : Constant  OutDataTypeStr=boolean
  Relational Operator : RelationalOperator  Operator=~=  OutDataTypeStr=boolean  RndMeth=Simplest
  Relational Operator1 : RelationalOperator  Operator===  OutDataTypeStr=boolean  RndMeth=Simplest
  Unit Delay : UnitDelay  SampleTime=-1
  Out1 : Outport
  wires:
  In1/1 -> Relational Operator1/2, Relational Operator/1, Unit Delay/1
  Unit Delay/1 -> Relational Operator/2
  Relational Operator/1 -> AND/2
  Constant/1 -> Relational Operator1/1
  Relational Operator1/1 -> AND/1
  AND/1 -> Out1/1

== system ModeStatAndRsp/ModeStatAndRsp_Runnable_sys/Subsystem1/Subsystem/HasChangeToTrue7 ==
  In1 : Inport
  AND : Logic  AllPortsSameDT=off  OutDataTypeStr=boolean
  Constant : Constant  OutDataTypeStr=boolean
  Relational Operator : RelationalOperator  Operator=~=  OutDataTypeStr=boolean  RndMeth=Simplest
  Relational Operator1 : RelationalOperator  Operator===  OutDataTypeStr=boolean  RndMeth=Simplest
  Unit Delay : UnitDelay  SampleTime=-1
  Out1 : Outport
  wires:
  AND/1 -> Out1/1
  Relational Operator1/1 -> AND/1
  Constant/1 -> Relational Operator1/1
  Relational Operator/1 -> AND/2
  Unit Delay/1 -> Relational Operator/2
  In1/1 -> Unit Delay/1, Relational Operator/1, Relational Operator1/2

== system ModeStatAndRsp/ModeStatAndRsp_Runnable_sys/Subsystem1/Subsystem/HasChangeToTrue8 ==
  In1 : Inport
  AND : Logic  AllPortsSameDT=off  OutDataTypeStr=boolean
  Constant : Constant  OutDataTypeStr=boolean
  Relational Operator : RelationalOperator  Operator=~=  OutDataTypeStr=boolean  RndMeth=Simplest
  Relational Operator1 : RelationalOperator  Operator===  OutDataTypeStr=boolean  RndMeth=Simplest
  Unit Delay : UnitDelay  SampleTime=-1
  Out1 : Outport
  wires:
  In1/1 -> Relational Operator1/2, Relational Operator/1, Unit Delay/1
  Unit Delay/1 -> Relational Operator/2
  Relational Operator/1 -> AND/2
  Constant/1 -> Relational Operator1/1
  Relational Operator1/1 -> AND/1
  AND/1 -> Out1/1

== system ModeStatAndRsp/ModeStatAndRsp_Runnable_sys/Subsystem1/Subsystem/HasChangeToTrue9 ==
  In1 : Inport
  AND : Logic  AllPortsSameDT=off  OutDataTypeStr=boolean
  Constant : Constant  OutDataTypeStr=boolean
  Relational Operator : RelationalOperator  Operator=~=  OutDataTypeStr=boolean  RndMeth=Simplest
  Relational Operator1 : RelationalOperator  Operator===  OutDataTypeStr=boolean  RndMeth=Simplest
  Unit Delay : UnitDelay  SampleTime=-1
  Out1 : Outport
  wires:
  AND/1 -> Out1/1
  Relational Operator1/1 -> AND/1
  Constant/1 -> Relational Operator1/1
  Relational Operator/1 -> AND/2
  Unit Delay/1 -> Relational Operator/2
  In1/1 -> Unit Delay/1, Relational Operator/1, Relational Operator1/2

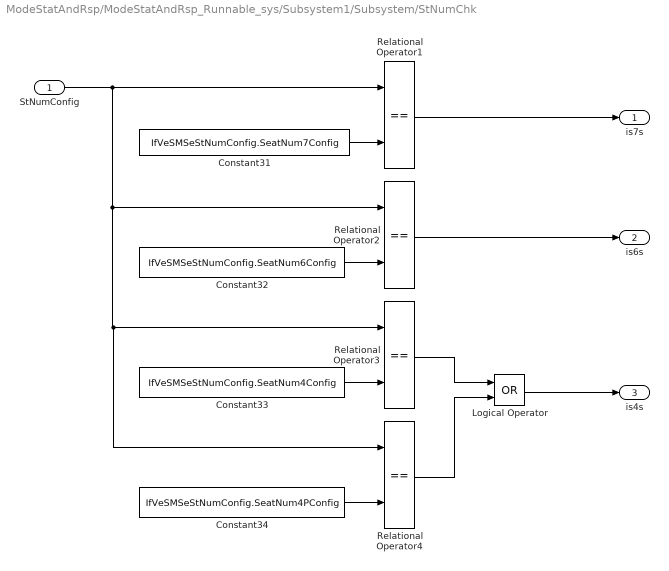
== system ModeStatAndRsp/ModeStatAndRsp_Runnable_sys/Subsystem1/Subsystem/StNumChk ==
  StNumConfig : Inport
  Constant31 : Constant  Value=IfVeSMSeStNumConfig.SeatNum7Config  OutDataTypeStr=Enum: IfVeSMSeStNumConfig
  Constant32 : Constant  Value=IfVeSMSeStNumConfig.SeatNum6Config  OutDataTypeStr=Enum: IfVeSMSeStNumConfig
  Constant33 : Constant  Value=IfVeSMSeStNumConfig.SeatNum4Config  OutDataTypeStr=Enum: IfVeSMSeStNumConfig
  Constant34 : Constant  Value=IfVeSMSeStNumConfig.SeatNum4PConfig  OutDataTypeStr=Enum: IfVeSMSeStNumConfig
  Logical Operator : Logic  Operator=OR  AllPortsSameDT=off  OutDataTypeStr=boolean
  Relational Operator{1..4} (4 alike) : RelationalOperator  Operator===  OutDataTypeStr=boolean  RndMeth=Simplest
  is7s : Outport
  is6s : Outport  Port=2
  is4s : Outport  Port=3
  wires:
  Constant34/1 -> Relational Operator4/2
  StNumConfig/1 -> Relational Operator1/1, Relational Operator4/1, Relational Operator3/1, Relational Operator2/1
  Logical Operator/1 -> is4s/1
  Relational Operator2/1 -> is6s/1
  Constant32/1 -> Relational Operator2/2
  Relational Operator1/1 -> is7s/1
  Relational Operator4/1 -> Logical Operator/2
  Relational Operator3/1 -> Logical Operator/1
  Constant31/1 -> Relational Operator1/2
  Constant33/1 -> Relational Operator3/2

== stateflow chart ModeStatAndRsp/ModeStatAndRsp_Runnable_sys/Subsystem1/FeedbackModeStatAndRsp/Subsystem3/Chart ==
  (default) -> (junction 5) : {i=0;}
  (junction 7) -> (junction 22) [order 1] : [PosArray[i+1]<1]
  (junction 5) -> (junction 7) [order 1] : [i<KeSMSbSRSPosNumConfig]
  (junction 7) -> (junction 9) [order 2] : {
      | ModeStatSRSswArray[i]=ModeStatArray[PosArray[i+1]-1];
      | }
  (junction 22) -> (junction 24) : {
      | ModeStatSRSswArray[i]=0;
      | }
  (junction 9) -> (junction 5) : {i=i+1;}
  (junction 5) -> (junction 12) [order 2]
  (junction 24) -> (junction 9)
  (junction 12) -> (junction 14) [order 1] : [i<10]
  (junction 14) -> (junction 16) : {
      | ModeStatSRSswArray[i]=0;
      | }
  (junction 16) -> (junction 12) : {i=i+1;}
  (junction 12) -> (junction 19) [order 2]
  data: ModeStatArray input uint8 size=32; KeSMSbSRSPosNumConfig input uint8; i local uint8; ModeStatSRSswArray output uint8 size=10; PosArray input uint8 size=11
